simulink model "VehicleDynamics_Test_Template"  (R2022b)
settings: Solver=VariableStepAuto  StartTime=0.0  StopTime=130  RelTol=1e-3  EnableMultiTasking=on
undefined symbols (not defined in the file): b, DiscIntNeverNeededParam, m
libraries: simulink x1
settings Model: Creator=raoulkumar  LastModifiedBy=abernjoh
settings SolverCC: AlgebraicLoopSolver=TrustRegion
settings DataIOCC: LimitDataPoints=on  ReturnWorkspaceOutputs=off
settings OptimizationCC: LifeSpan=inf
settings DebuggingCC: UnconnectedInputMsg=warning  UnconnectedOutputMsg=warning  UnconnectedLineMsg=warning  AllowSymbolicDim=off  SFUnexpectedBacktrackingDiag=warning  SFNoUnconditionalDefaultTransitionDiag=warning  SFExecutionAtInitializationDiag=none  SFMachineParentedDataDiag=warning  ArithmeticOperatorsInVariantConditions=warning
settings ModelReferenceCC: EnableRefExpFcnMdlSchedulingChecks=on  PropagateSignalLabelsOutOfModel=off
settings SFSimCC: SimUseLocalCustomCode=off  CustomCodeUndefinedFunction=UseInterfaceOnly
settings RTWCC: RTWUseLocalCustomCode=off
settings CodeAppCC: StateflowObjectComments=on
settings GRTTargetCC: TargetLangStandard=C89/C90 (ANSI)
settings ConfigComp: CovMetricSettings=dw  CovSaveCumulativeToWorkspaceVar=on  CovSaveSingleToWorkspaceVar=on  CovExternalEMLEnable=off

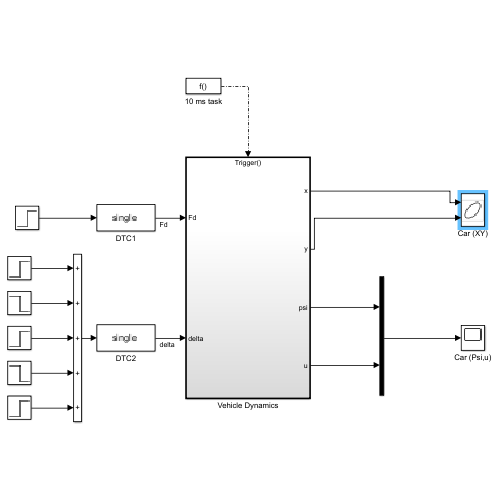
[thumbnail: Simulink's stored preview of the top-level diagram]
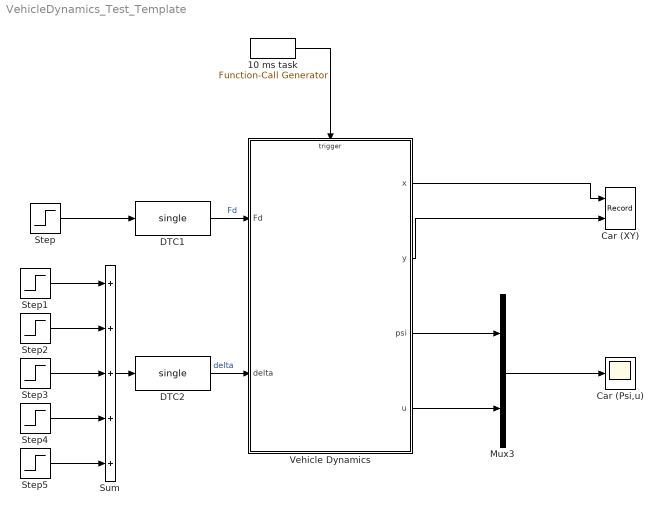
== system VehicleDynamics_Test_Template ==
  10 ms task : simulink/Ports & Subsystems/Function-Call Generator  sample_time=0.01  numberOfIterations=1  DisallowWideOutput=off
  Car (Psi,u) : Scope
  Car (XY) : Record  FileSettingsInternal="{\"entries\":[{\"content\":{\"excelSettings\":{\"content\":{},\"type\":\"Streamout.ExcelSettings\"}},\"type\":\"Streamout.FileSettingStorage\",\"uuid\":\"2b865681-a899-4e4e-b0df-2d0dc68b4d00\"}],\"packageUris\":[\"http://schema.mathworks.com/mf0/streamout_blocks/R2020a\"],\"version\":\"1.0\"}"  Layout=[1 1]  SignalsInternal="{\"entries\":[{\"content\":{\"signals\":[{\"content\":{\"blockPath\":[\"VehicleDynamics_Test_Template/Car (XY)\"],\"channel\":[],\"dimensions\":[1],\"domain\":\"VehicleDynamics_Test_Template/Car (XY)\",\"lineColor\":\"#a2142f\",\"plots\":[1],\"port\":1,\"sid\":[\"\"],\"signalID\":55,\"signalName\":\"Vehicle Dynamics:1\"},\"type\":\"RecordBlkView.Signal\",\"uuid\":\"fba3bb43-f7c2-4683-9da4-2a2f48e8d9b2\"},{\"content\":{\"blockPath\":[\"VehicleDynamics_Test_Template/Car (XY)\"],\"channel\":[],\"dimensions\":[1],\"domain\":\"VehicleDynamics_Test_Template/Car (XY)\",\"lineColor\":\"#139fff\",\"plots\":[1],\"port\":2,\"sid\":[\"\"],\"signalID\":59,\"signalName\":\"Vehicle Dynamics:2\"},\"type\":\"RecordBlkView.Signal\",\"uuid\":\"ab60afc6-4eb8-4b9b-a313-8ba0df7f8c3b\"}]},\"type\":\"RecordBlkView.InputSignals\",\"uuid\":\"919faf4d-fc62-432e-84d3-92c11d7f8a70\"}],\"packageUris\":[\"http://schema.mathworks.com/mf0/streamout_blocks/R2020a\"],\"version\":\"1.0\"}"  VisualizationBindings="{\"xyplotplugin\":{\"info\":[{\"series\":[{\"bindingParametersList\":[{\"parameter\":\"X-Axis\",\"signalID\":55,\"signalName\":\"Vehicle Dynamics:1\"},{\"parameter\":\"Y-Axis\",\"signalID\":59,\"signalName\":\"Vehicle Dynamics:2\"}],\"seriesID\":20899}],\"subplotID\":1}]}}"  CompatibilityTag=XY  st=-1
  DTC1 : DataTypeConversion  OutDataTypeStr=single  SaturateOnIntegerOverflow=off  RndMeth=Floor
  DTC2 : DataTypeConversion  OutDataTypeStr=single  SaturateOnIntegerOverflow=off  RndMeth=Floor
  Mux3 : Mux  Inputs=2
  Step : Step  After=1000
  Step1 : Step  Time=30  After=2*pi/180
  Step2 : Step  Time=50  After=-4*pi/180
  Step3 : Step  Time=70  After=5*pi/180
  Step4 : Step  Time=83  After=-3*pi/180
  Step5 : Step  Time=110  After=0.7*pi/180
  Sum : Sum  Inputs=+++++
  Vehicle Dynamics : Subsystem  TreatAsAtomicUnit=on
  wires:
  10 ms task/1 -> Vehicle Dynamics/Trigger
  Vehicle Dynamics/1(x) -> Car (XY)/1
  Vehicle Dynamics/2(y) -> Car (XY)/2
  Mux3/1 -> Car (Psi,u)/1
  Step/1 -> DTC1/1
  Sum/1 -> DTC2/1
  Step1/1 -> Sum/1
  Step2/1 -> Sum/2
  Step3/1 -> Sum/3
  Step4/1 -> Sum/4
  Step5/1 -> Sum/5
  DTC1/1 -> Vehicle Dynamics/1(Fd)  "Fd"
  DTC2/1 -> Vehicle Dynamics/2(delta)  "delta"
  Vehicle Dynamics/3(psi) -> Mux3/1
  Vehicle Dynamics/4(u) -> Mux3/2

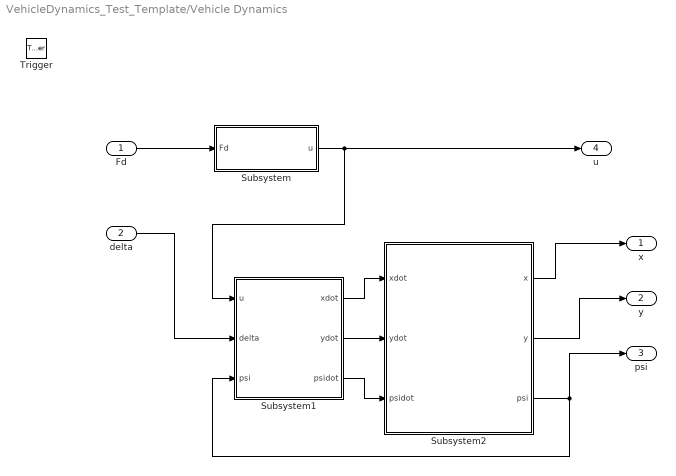
== system VehicleDynamics_Test_Template/Vehicle Dynamics ==
  Fd : Inport
  delta : Inport  Port=2
  Trigger : TriggerPort  TriggerType=function-call  VariantControl=(inherit)
  Subsystem : Subsystem
  Subsystem1 : Subsystem
  Subsystem2 : Subsystem
  x : Outport
  y : Outport  Port=2
  psi : Outport  Port=3
  u : Outport  Port=4
  wires:
  Fd/1 -> Subsystem/1(Fd)
  delta/1 -> Subsystem1/2(delta)
  Subsystem2/1(x) -> x/1
  Subsystem2/2(y) -> y/1
  Subsystem2/3(psi) -> psi/1, Subsystem1/3(psi)
  Subsystem/1(u) -> Subsystem1/1(u), u/1
  Subsystem1/3(psidot) -> Subsystem2/3(psidot)
  Subsystem1/2(ydot) -> Subsystem2/2(ydot)
  Subsystem1/1(xdot) -> Subsystem2/1(xdot)

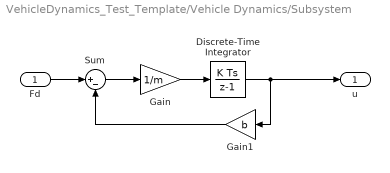
== system VehicleDynamics_Test_Template/Vehicle Dynamics/Subsystem ==
  Fd : Inport
  Discrete-Time Integrator : DiscreteIntegrator  gainval=1  SampleTime=-1  ICPrevOutput=DiscIntNeverNeededParam  ICPrevScaledInput=DiscIntNeverNeededParam
  Gain : Gain  Gain=1/m
  Gain1 : Gain  Gain=b
  Sum : Sum  Inputs=|+-
  u : Outport
  wires:
  Sum/1 -> Gain/1
  Fd/1 -> Sum/1
  Discrete-Time Integrator/1 -> Gain1/1, u/1
  Gain/1 -> Discrete-Time Integrator/1
  Gain1/1 -> Sum/2

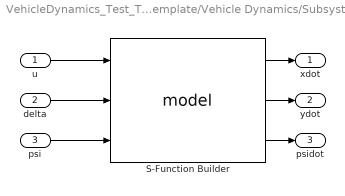
== system VehicleDynamics_Test_Template/Vehicle Dynamics/Subsystem1 ==
  u : Inport
  delta : Inport  Port=2
  psi : Inport  Port=3
  S-Function Builder : S-Function  FunctionName=model  Parameters=single(1),single(1)  SFunctionModules=model_wrapper  SFunctionDeploymentMode=off  EnableBusSupport=off  mask(S-Function Builder){}
      mask help: Simulink:masks:SFunctionBuilder_MD
      mask init:
      | val = [[.9  0.75 0.75 1 1 .9 .9 1]',[1 1 0.75 0.75 .9 .9 1 .9]'];try , sys = get_param(gcb,'SfunBuilderFcnName');if isempty(sys), sys = get_param(gcb,'FunctionName'); end,catch, sys = get_param(gcb,'FunctionName'); end
      settings: CopyFcn=set_param(gcbh,'LinkStatus','none')  OpenFcn=sfunctionwizard(gcbh)
      mask Display:
      | plot(val(:,1),val(:,2))
      | disp(sys)
      | port_label('input',1,'u')
      | port_label('input',2,'delta')
      | port_label('input',3,'psi')
      | port_label('output',1,'xdot')
      | port_label('output',2,'ydot')
      | port_label('output',3,'psidot')
  xdot : Outport
  ydot : Outport  Port=2
  psidot : Outport  Port=3
  wires:
  u/1 -> S-Function Builder/1
  delta/1 -> S-Function Builder/2
  psi/1 -> S-Function Builder/3
  S-Function Builder/1 -> xdot/1
  S-Function Builder/2 -> ydot/1
  S-Function Builder/3 -> psidot/1

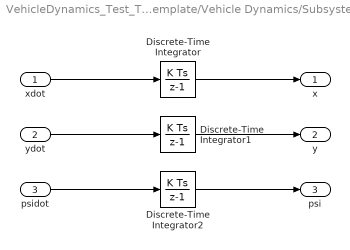
== system VehicleDynamics_Test_Template/Vehicle Dynamics/Subsystem2 ==
  xdot : Inport
  ydot : Inport  Port=2
  psidot : Inport  Port=3
  Discrete-Time Integrator : DiscreteIntegrator  SampleTime=-1  ICPrevOutput=DiscIntNeverNeededParam  ICPrevScaledInput=DiscIntNeverNeededParam
  Discrete-Time Integrator1 : DiscreteIntegrator  SampleTime=-1  ICPrevOutput=DiscIntNeverNeededParam  ICPrevScaledInput=DiscIntNeverNeededParam
  Discrete-Time Integrator2 : DiscreteIntegrator  SampleTime=-1  ICPrevOutput=DiscIntNeverNeededParam  ICPrevScaledInput=DiscIntNeverNeededParam
  x : Outport
  y : Outport  Port=2
  psi : Outport  Port=3
  wires:
  psidot/1 -> Discrete-Time Integrator2/1
  ydot/1 -> Discrete-Time Integrator1/1
  xdot/1 -> Discrete-Time Integrator/1
  Discrete-Time Integrator/1 -> x/1
  Discrete-Time Integrator1/1 -> y/1
  Discrete-Time Integrator2/1 -> psi/1
